simulink subsystem "Find_Target_Position_Velocity_Heading"  (R2023b)
settings: Solver=VariableStepAuto  StartTime=0.0  StopTime=10.0  RelTol=1e-3
undefined symbols (not defined in the file): Spline_Last_Pose_Distance_to_Velocity_Gain, Spline_Max_Centripital_Acceleration, Spline_Max_Num_RefPoses, Spline_Num_Samples, Spline_Pose_Num_Before_End_Reduce_Speed, Spline_Velocity_Multiplier_TEST
libraries: simulink x3
settings Model: Creator=ander  LastModifiedBy=ander

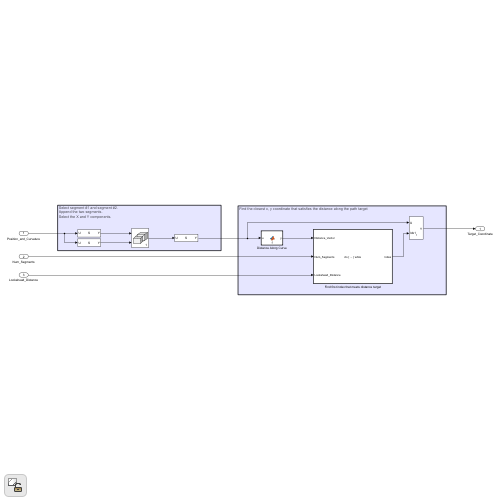
[thumbnail: Simulink's stored preview of the top-level diagram]
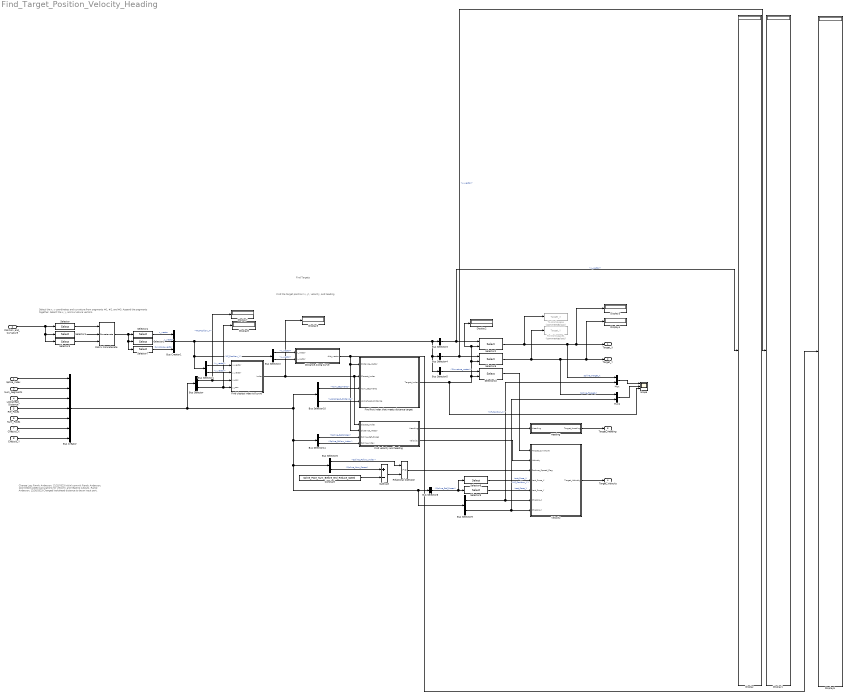
== system Find_Target_Position_Velocity_Heading ==
  note: Find the target position (x, y), velocity, and heading
  note: Select the x, y coordinates and curvature from segments #1, #2, and #3.
      | Append the segments together.
      | Select the x, y, and curvature vectors.
  note: Find Targets
  note: Change Log:
      | Randy Anderson: 12/25/2023
      | Initial commit
      | Randy Anderson, 12/27/2023
      | Added calculations for velocity and heading outputs.
      | Randy Anderson, 12/30/2023
      | Changed lookahead distance to be an input port.
  Spline_Index : Inport
  Position_and_Curvature : Inport  Port=2
  Num_Segments : Inport  Port=3
  Lookahead_Distance : Inport  Port=4  OutDataTypeStr=double  PortDimensions=1
  Ref_Poses : Inport  Port=5  OutDataTypeStr=double
  Num_Poses : Inport  Port=6
  Chassis_X : Inport  Port=7  OutDataTypeStr=double  PortDimensions=1
  Chassis_Y : Inport  Port=8  OutDataTypeStr=double  PortDimensions=1
  Bus Creator : BusCreator  Inputs=7
  Bus Creator1 : BusCreator  Inputs=3
  Bus Selector : BusSelector  OutputSignals=KF_Position_X,KF_Position_Y
  Bus Selector1 : BusSelector  OutputSignals=x_vector,y_vector
  Bus Selector10 : BusSelector  OutputSignals=Num_Segments,Lookahead_Distance
  Bus Selector11 : BusSelector  OutputSignals=Spline_Ref_Poses,Spline_Follow_Index
  Bus Selector2 : BusSelector  OutputSignals=x_vector,y_vector
  Bus Selector3 : BusSelector  OutputSignals=x_vector
  Bus Selector4 : BusSelector  OutputSignals=y_vector
  Bus Selector5 : BusSelector  OutputSignals=Curvature_vector
  Bus Selector6 : BusSelector  OutputSignals=Spline_Follow_Index,Spline_Num_Poses
  Bus Selector8 : BusSelector  OutputSignals=Spline_Ref_Poses
  Bus Selector9 : BusSelector  OutputSignals=KF_Position_X,KF_Position_Y
  Constant : Constant  Value=Spline_Pose_Num_Before_End_Reduce_Speed
  Display{,1..8} (9 alike) : Display
  Distance Along Curve : MATLAB Function  TreatAsAtomicUnit=on
  Find closest index to curve : MATLAB Function  TreatAsAtomicUnit=on
  Find first index that meets distance target : Subsystem  TreatAsAtomicUnit=on
  Find velocity and heading : Subsystem
  Heading : Subsystem
  Matrix Concatenate : Concatenate  NumInputs=3  Mode=Multidimensional array
  Mux : Mux  Inputs=2
  Mux1 : Mux  Inputs=2
  Relational Operator : RelationalOperator  OutDataTypeStr=boolean  RndMeth=Simplest  InputSameDT=off
  Scope : Scope  NumInputPorts=3
  Selector : Selector  NumberOfDimensions=3  InputPortWidth=3  IndexOptions=Select all,Select all,Index vector (dialog)  Indices=[1 3],[1 2],1  OutputSizes=1,1,1
  Selector1 : Selector  NumberOfDimensions=3  InputPortWidth=3  IndexOptions=Select all,Select all,Index vector (dialog)  Indices=[1 3],[1 2],2  OutputSizes=1,1,1
  Selector10 : Selector  InputPortWidth=Spline_Num_Samples_3x  IndexOptions=Index vector (port)  Indices=[1 3]  OutputSizes=1
  Selector2 : Selector  InputPortWidth=Spline_Num_Samples_3x  IndexOptions=Index vector (port)  Indices=[1 3]  OutputSizes=1
  Selector3 : Selector  NumberOfDimensions=3  InputPortWidth=3  IndexOptions=Select all,Select all,Index vector (dialog)  Indices=[1 3],[1 2],3  OutputSizes=1,1,1
  Selector4 : Selector  NumberOfDimensions=2  InputPortWidth=3  IndexOptions=Select all,Index vector (dialog)  Indices=[1 3],1  OutputSizes=1,1
  Selector5 : Selector  NumberOfDimensions=2  InputPortWidth=3  IndexOptions=Select all,Index vector (dialog)  Indices=[1 3],2  OutputSizes=1,1
  Selector6 : Selector  InputPortWidth=Spline_Num_Samples_3x  IndexOptions=Index vector (port)  Indices=[1 3]  OutputSizes=1
  Selector7 : Selector  NumberOfDimensions=2  InputPortWidth=3  IndexOptions=Select all,Index vector (dialog)  Indices=[1 3],3  OutputSizes=1,1
  Selector8 : Selector  NumberOfDimensions=2  InputPortWidth=3  IndexOptions=Index vector (dialog),Index vector (dialog)  Indices=Spline_Max_Num_RefPoses,1  OutputSizes=1,1
  Selector9 : Selector  NumberOfDimensions=2  InputPortWidth=3  IndexOptions=Index vector (dialog),Index vector (dialog)  Indices=Spline_Max_Num_RefPoses,2  OutputSizes=1,1
  Subtract : Sum  Inputs=+-
  To Workspace : ToWorkspace  Commented=on  VariableName=Target_X  SampleTime=-1
  To Workspace1 : ToWorkspace  Commented=on  VariableName=Target_Y  SampleTime=-1
  Velocity : Subsystem
  Target_X : Outport
  Target_Y : Outport  Port=2
  Target_Heading : Outport  Port=3
  Target_Velocity : Outport  Port=4
  wires:
  Selector1/1 -> Matrix Concatenate/2
  Matrix Concatenate/1 -> Selector4/1, Selector5/1, Selector7/1
  Selector/1 -> Matrix Concatenate/1
  Distance Along Curve/1(dist_vector) -> Find first index that meets distance target/1(Distance_Vector), Find velocity and heading/2(Distance_Vector), Display6/1
  Selector3/1 -> Matrix Concatenate/3
  Bus Creator/1 -> Bus Selector11/1, Bus Selector9/1, Bus Selector8/1, Bus Selector6/1, Bus Selector10/1, Bus Selector/1
  Selector5/1 -> Bus Creator1/2  "y_vector"
  Selector4/1 -> Bus Creator1/1  "x_vector"
  Bus Creator1/1 -> Bus Selector3/1, Bus Selector4/1, Bus Selector5/1, Bus Selector2/1, Bus Selector1/1
  Bus Selector1/1 -> Find closest index to curve/1(x_vector)  "<x_vector>"
  Bus Selector1/2 -> Find closest index to curve/2(y_vector)  "<y_vector>"
  Bus Selector/2 -> Find closest index to curve/4(y_pos), Display8/1  "<KF_Position_Y>"
  Bus Selector/1 -> Find closest index to curve/3(x_pos), Display7/1  "<KF_Position_X>"
  Bus Selector2/2 -> Distance Along Curve/2(y_vector)  "<y_vector>"
  Bus Selector2/1 -> Distance Along Curve/1(x_vector)  "<x_vector>"
  Bus Selector3/1 -> Selector2/1, Display/1  "<x_vector>"
  Bus Selector4/1 -> Selector6/1, Display1/1  "<y_vector>"
  Selector2/1 -> To Workspace/1, Target_X/1, Display3/1, Mux/1  "Spline_Target_X"
  Selector6/1 -> To Workspace1/1, Target_Y/1, Display4/1, Mux1/1  "Spline_Target_Y"
  Bus Selector10/2 -> Find first index that meets distance target/4(Lookahead_Distance)  "<Lookahead_Distance>"
  Position_and_Curvature/1 -> Selector/1, Selector1/1, Selector3/1
  Selector10/1 -> Velocity/1(Target_Curvature)
  Bus Selector5/1 -> Selector10/1  "<Curvature_vector>"
  Find first index that meets distance target/1(Target_Index) -> Display2/1, Selector2/2, Selector6/2, Selector10/2, Scope/3
  Selector7/1 -> Bus Creator1/3  "Curvature_vector"
  Constant/1 -> Subtract/2
  Subtract/1 -> Relational Operator/2
  Selector8/1 -> Velocity/4(Last_Pose_X)  "Last_Pose_X"
  Selector9/1 -> Velocity/5(Last_Pose_Y)  "Last_Pose_Y"
  Relational Operator/1 -> Velocity/3(Reduce_Speed_Flag)
  Velocity/1(Target_Velocity) -> Target_Velocity/1
  Bus Selector6/1 -> Relational Operator/1  "<Spline_Follow_Index>"
  Bus Selector8/1 -> Selector9/1, Selector8/1  "<Spline_Ref_Poses>"
  Bus Selector9/1 -> Velocity/6(Chassis_X), Mux/2  "<KF_Position_X>"
  Bus Selector9/2 -> Velocity/7(Chassis_Y), Mux1/2  "<KF_Position_Y>"
  Bus Selector10/1 -> Find first index that meets distance target/3(Num_Segments)  "<Num_Segments>"
  Spline_Index/1 -> Bus Creator/1
  Num_Segments/1 -> Bus Creator/2
  Ref_Poses/1 -> Bus Creator/4
  Num_Poses/1 -> Bus Creator/5
  Chassis_X/1 -> Bus Creator/6
  Chassis_Y/1 -> Bus Creator/7
  Heading/1(Target_Heading) -> Target_Heading/1
  Bus Selector6/2 -> Subtract/1  "<Spline_Num_Poses>"
  Find closest index to curve/1(index) -> Find first index that meets distance target/2(Closest_Index), Find velocity and heading/1(Closest_Index), Display5/1
  Bus Selector11/1 -> Find velocity and heading/3(Spline_Ref_Poses)  "<Spline_Ref_Poses>"
  Bus Selector11/2 -> Find velocity and heading/4(Spline_Index)  "<Spline_Follow_Index>"
  Find velocity and heading/2(Velocity) -> Velocity/2(Velocity)
  Find velocity and heading/1(Heading) -> Heading/1(Heading)
  Lookahead_Distance/1 -> Bus Creator/3
  Mux/1 -> Scope/1
  Mux1/1 -> Scope/2

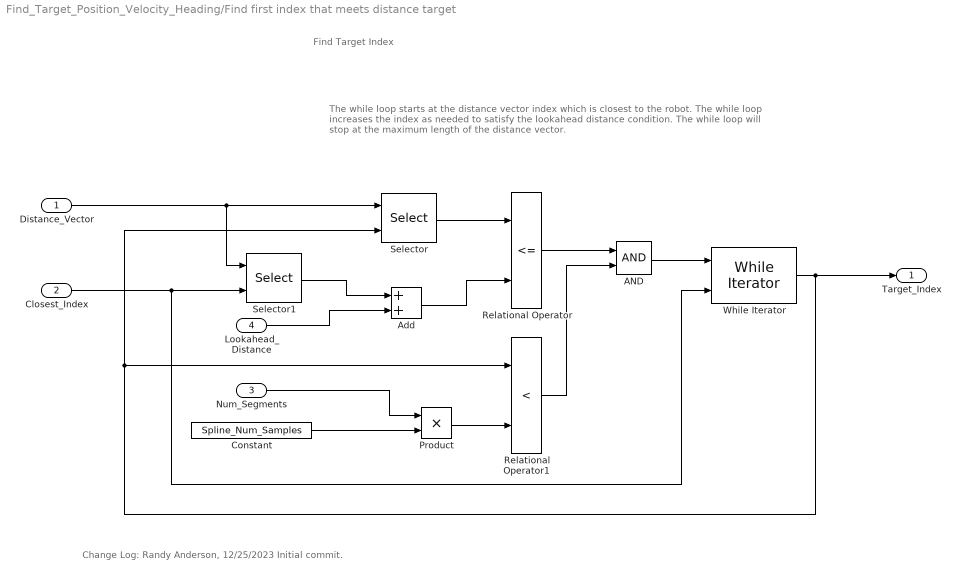
== system Find_Target_Position_Velocity_Heading/Find first index that meets distance target ==
  note: Change Log:
      | Randy Anderson, 12/25/2023
      | Initial commit.
  note: The while loop starts at the distance vector index which is closest to the robot.
      | The while loop increases the index as needed to satisfy the lookahead distance condition.
      | The while loop will stop at the maximum length of the distance vector.
  note: Find Target Index
  Distance_Vector : Inport
  Closest_Index : Inport  Port=2
  Num_Segments : Inport  Port=3
  Lookahead_Distance : Inport  Port=4
  AND : Logic  AllPortsSameDT=off  OutDataTypeStr=boolean
  Add : Sum
  Constant : Constant  Value=Spline_Num_Samples
  Product : Product
  Relational Operator : RelationalOperator  Operator=<=  OutDataTypeStr=boolean  RndMeth=Simplest  InputSameDT=off
  Relational Operator1 : RelationalOperator  Operator=<  OutDataTypeStr=boolean  RndMeth=Simplest  InputSameDT=off
  Selector : Selector  InputPortWidth=Spline_Num_Samples_3x  IndexOptions=Index vector (port)  Indices=[1 3]  OutputSizes=1
  Selector1 : Selector  InputPortWidth=Spline_Num_Samples_3x  IndexOptions=Index vector (port)  Indices=[1 3]  OutputSizes=1
  While Iterator : WhileIterator  MaxIters=Spline_Num_Samples_3x  ShowIterationPort=on  OutputDataType=uint16
  Target_Index : Outport
  wires:
  Selector1/1 -> Add/1
  Lookahead_Distance/1 -> Add/2
  Add/1 -> Relational Operator/2
  Closest_Index/1 -> Selector1/2, While Iterator/2
  AND/1 -> While Iterator/1
  Relational Operator/1 -> AND/1
  Relational Operator1/1 -> AND/2
  Constant/1 -> Product/2
  Num_Segments/1 -> Product/1
  Product/1 -> Relational Operator1/2
  While Iterator/1 -> Selector/2, Relational Operator1/1, Target_Index/1
  Selector/1 -> Relational Operator/1
  Distance_Vector/1 -> Selector/1, Selector1/1

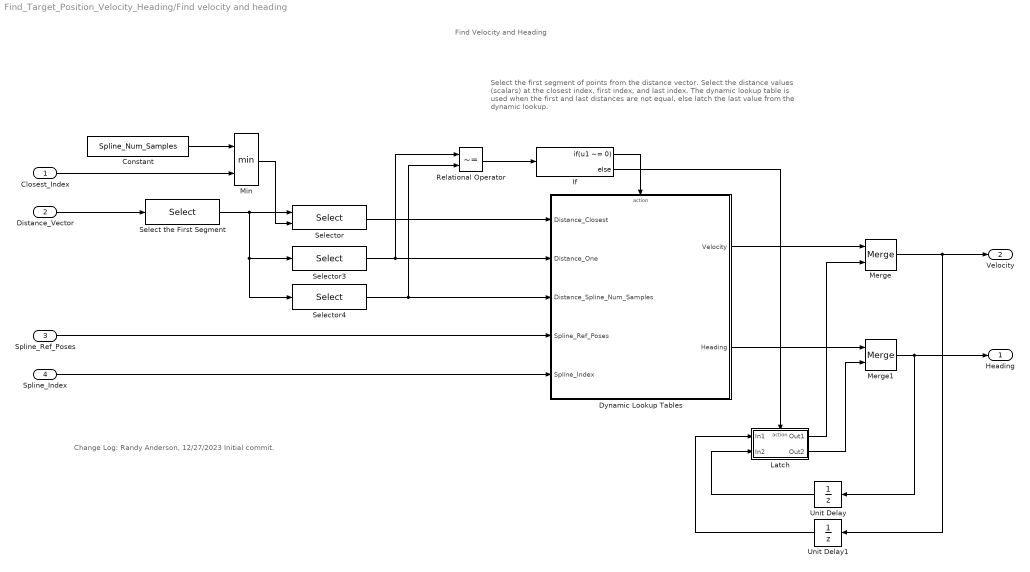
== system Find_Target_Position_Velocity_Heading/Find velocity and heading ==
  note: Change Log:
      | Randy Anderson, 12/27/2023
      | Initial commit.
  note: Find Velocity and Heading
  note: Select the first segment of points from the distance vector.
      | Select the distance values (scalars) at the closest index, first index, and last index.
      | The dynamic lookup table is used when the first and last distances are not equal,
      |    else latch the last value from the dynamic lookup.
  Closest_Index : Inport
  Distance_Vector : Inport  Port=2
  Spline_Ref_Poses : Inport  Port=3
  Spline_Index : Inport  Port=4
  Constant : Constant  Value=Spline_Num_Samples
  Dynamic Lookup Tables : Subsystem
  If : If  IfExpression=u1 ~= 0
  Latch : Subsystem  TreatAsAtomicUnit=on
  Merge : Merge
  Merge1 : Merge
  Min : MinMax  Inputs=2
  Relational Operator : RelationalOperator  Operator=~=  OutDataTypeStr=boolean  RndMeth=Simplest  InputSameDT=off
  Select the First Segment : Selector  InputPortWidth=Spline_Num_Samples_3x  IndexOptions=Index vector (dialog)  Indices=[1:Spline_Num_Samples]  OutputSizes=1
  Selector : Selector  InputPortWidth=Spline_Num_Samples  IndexOptions=Index vector (port)  Indices=[1:Spline_Num_Samples]  OutputSizes=1
  Selector3 : Selector  InputPortWidth=Spline_Num_Samples  IndexOptions=Index vector (dialog)  Indices=1  OutputSizes=1
  Selector4 : Selector  InputPortWidth=Spline_Num_Samples  IndexOptions=Index vector (dialog)  Indices=Spline_Num_Samples  OutputSizes=1
  Unit Delay : UnitDelay  SampleTime=-1  HasFrameUpgradeWarning=on
  Unit Delay1 : UnitDelay  SampleTime=-1  HasFrameUpgradeWarning=on
  Heading : Outport
  Velocity : Outport  Port=2
  wires:
  Constant/1 -> Min/1
  Min/1 -> Selector/2
  Unit Delay1/1 -> Latch/1(In1)
  Unit Delay/1 -> Latch/2(In2)
  Merge/1 -> Velocity/1, Unit Delay1/1
  Merge1/1 -> Unit Delay/1, Heading/1
  Latch/2(Out2) -> Merge1/2
  Dynamic Lookup Tables/2(Heading) -> Merge1/1
  Latch/1(Out1) -> Merge/2
  Dynamic Lookup Tables/1(Velocity) -> Merge/1
  If/2 -> Latch/Action
  If/1 -> Dynamic Lookup Tables/Action
  Spline_Index/1 -> Dynamic Lookup Tables/5(Spline_Index)
  Spline_Ref_Poses/1 -> Dynamic Lookup Tables/4(Spline_Ref_Poses)
  Selector/1 -> Dynamic Lookup Tables/1(Distance_Closest)
  Relational Operator/1 -> If/1
  Selector4/1 -> Dynamic Lookup Tables/3(Distance_Spline_Num_Samples), Relational Operator/2
  Select the First Segment/1 -> Selector/1, Selector3/1, Selector4/1
  Selector3/1 -> Dynamic Lookup Tables/2(Distance_One), Relational Operator/1
  Closest_Index/1 -> Min/2
  Distance_Vector/1 -> Select the First Segment/1

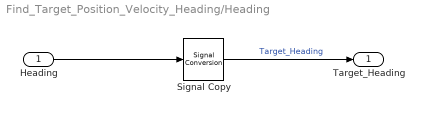
== system Find_Target_Position_Velocity_Heading/Heading ==
  Heading : Inport
  Signal Copy : SignalConversion  OverrideOpt=off
  Target_Heading : Outport
  wires:
  Heading/1 -> Signal Copy/1
  Signal Copy/1 -> Target_Heading/1  "Target_Heading"

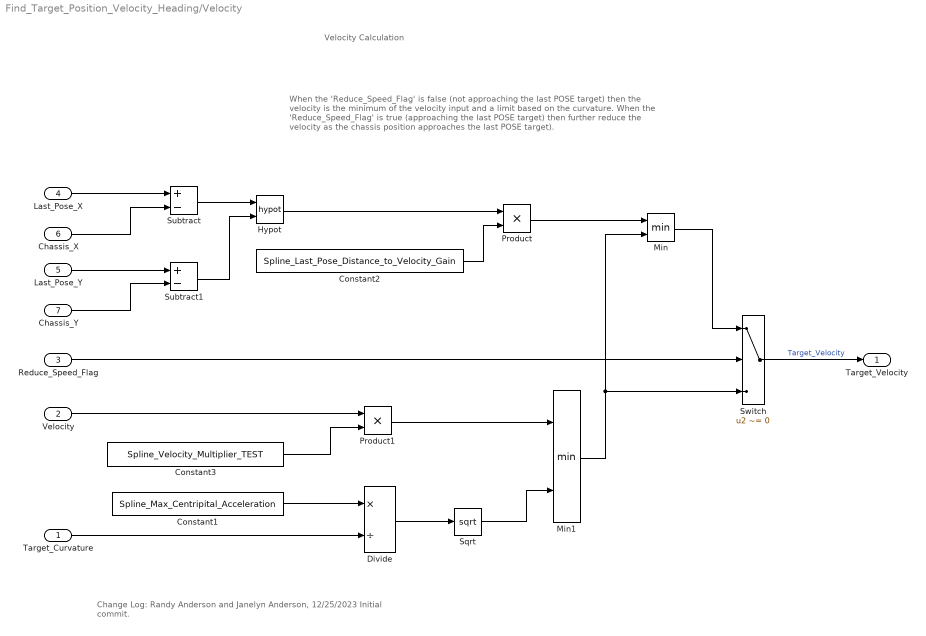
== system Find_Target_Position_Velocity_Heading/Velocity ==
  note: When the 'Reduce_Speed_Flag' is false (not approaching the last POSE target) then
      | the velocity is the minimum of the velocity input and a limit based on the curvature.
      |
      | When the 'Reduce_Speed_Flag' is true (approaching the last POSE target) then further
      | reduce the velocity as the chassis position approaches the last POSE target).
  note: Velocity Calculation
  note: Change Log:
      | Randy Anderson and Janelyn Anderson, 12/25/2023
      | Initial commit.
  Target_Curvature : Inport
  Velocity : Inport  Port=2
  Reduce_Speed_Flag : Inport  Port=3
  Last_Pose_X : Inport  Port=4
  Last_Pose_Y : Inport  Port=5
  Chassis_X : Inport  Port=6  OutDataTypeStr=double  PortDimensions=1
  Chassis_Y : Inport  Port=7  OutDataTypeStr=double  PortDimensions=1
  Constant1 : Constant  Value=Spline_Max_Centripital_Acceleration
  Constant2 : Constant  Value=Spline_Last_Pose_Distance_to_Velocity_Gain
  Constant3 : Constant  Value=Spline_Velocity_Multiplier_TEST
  Divide : Product  Inputs=*/
  Hypot : Math  Operator=hypot
  Min : MinMax  Inputs=2
  Min1 : MinMax  Inputs=2
  Product : Product
  Product1 : Product
  Sqrt : Sqrt
  Subtract : Sum  Inputs=+-
  Subtract1 : Sum  Inputs=+-
  Switch : Switch  Criteria=u2 ~= 0  SaturateOnIntegerOverflow=off  InputSameDT=off
  Target_Velocity : Outport
  wires:
  Constant3/1 -> Product1/2
  Velocity/1 -> Product1/1
  Product1/1 -> Min1/1
  Switch/1 -> Target_Velocity/1  "Target_Velocity"
  Constant2/1 -> Product/2
  Product/1 -> Min/1
  Hypot/1 -> Product/1
  Sqrt/1 -> Min1/2
  Divide/1 -> Sqrt/1
  Constant1/1 -> Divide/1
  Target_Curvature/1 -> Divide/2
  Min/1 -> Switch/1
  Reduce_Speed_Flag/1 -> Switch/2
  Min1/1 -> Switch/3, Min/2
  Subtract1/1 -> Hypot/2
  Subtract/1 -> Hypot/1
  Chassis_Y/1 -> Subtract1/2
  Last_Pose_Y/1 -> Subtract1/1
  Chassis_X/1 -> Subtract/2
  Last_Pose_X/1 -> Subtract/1

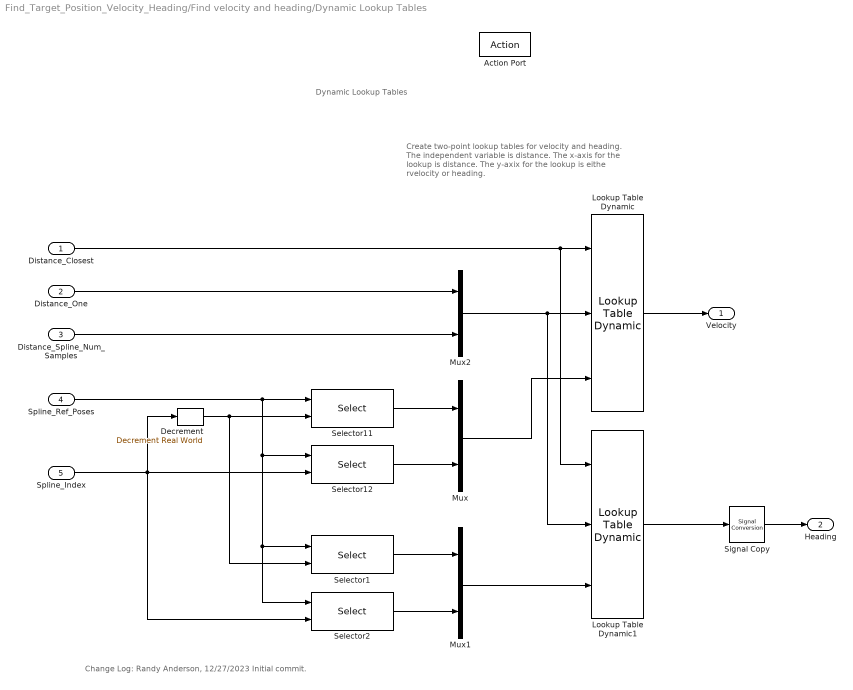
== system Find_Target_Position_Velocity_Heading/Find velocity and heading/Dynamic Lookup Tables ==
  note: Change Log:
      | Randy Anderson, 12/27/2023
      | Initial commit.
  note: Dynamic Lookup Tables
  note: Create two-point lookup tables for velocity and heading.
      | The independent variable is distance.
      | The x-axis for the lookup is distance.
      | The y-axix for the lookup is eithe rvelocity or heading.
  Distance_Closest : Inport
  Distance_One : Inport  Port=2
  Distance_Spline_Num_Samples : Inport  Port=3
  Spline_Ref_Poses : Inport  Port=4
  Spline_Index : Inport  Port=5
  Action Port : ActionPort
  Decrement : simulink/Additional Math & Discrete/Additional Math: Increment - Decrement/Decrement Real World
  Lookup Table Dynamic : simulink/Lookup Tables/Lookup Table Dynamic  LookUpMeth=Interpolation-Use End Values  OutDataType=fixdt('double')  OutScaling=[]  OutputDataTypeScalingMode=Specify via dialog  OutDataTypeStr=double  DoSatur=off
  Lookup Table Dynamic1 : simulink/Lookup Tables/Lookup Table Dynamic  LookUpMeth=Interpolation-Use End Values  OutDataType=fixdt('double')  OutScaling=[]  OutputDataTypeScalingMode=Specify via dialog  OutDataTypeStr=double  DoSatur=off
  Mux : Mux  Inputs=2
  Mux1 : Mux  Inputs=2
  Mux2 : Mux  Inputs=2
  Selector1 : Selector  NumberOfDimensions=2  InputPortWidth=Spline_Num_Samples_x3  IndexOptions=Index vector (port),Index vector (dialog)  Indices=[1 3],4  OutputSizes=1,1
  Selector11 : Selector  NumberOfDimensions=2  InputPortWidth=Spline_Num_Samples_x3  IndexOptions=Index vector (port),Index vector (dialog)  Indices=[1 3],3  OutputSizes=1,1
  Selector12 : Selector  NumberOfDimensions=2  InputPortWidth=Spline_Num_Samples_x3  IndexOptions=Index vector (port),Index vector (dialog)  Indices=[1 3],3  OutputSizes=1,1
  Selector2 : Selector  NumberOfDimensions=2  InputPortWidth=Spline_Num_Samples_x3  IndexOptions=Index vector (port),Index vector (dialog)  Indices=[1 3],4  OutputSizes=1,1
  Signal Copy : SignalConversion  OverrideOpt=off
  Velocity : Outport
  Heading : Outport  Port=2
  wires:
  Signal Copy/1 -> Heading/1
  Mux/1 -> Lookup Table Dynamic/3
  Distance_One/1 -> Mux2/1
  Lookup Table Dynamic/1 -> Velocity/1
  Selector1/1 -> Mux1/1
  Selector11/1 -> Mux/1
  Distance_Spline_Num_Samples/1 -> Mux2/2
  Decrement/1 -> Selector1/2, Selector11/2
  Mux1/1 -> Lookup Table Dynamic1/3
  Selector2/1 -> Mux1/2
  Mux2/1 -> Lookup Table Dynamic/2, Lookup Table Dynamic1/2
  Spline_Index/1 -> Selector12/2, Selector2/2, Decrement/1
  Lookup Table Dynamic1/1 -> Signal Copy/1
  Spline_Ref_Poses/1 -> Selector12/1, Selector1/1, Selector2/1, Selector11/1
  Selector12/1 -> Mux/2
  Distance_Closest/1 -> Lookup Table Dynamic/1, Lookup Table Dynamic1/1

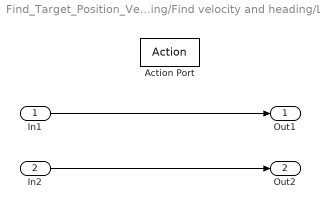
== system Find_Target_Position_Velocity_Heading/Find velocity and heading/Latch ==
  In1 : Inport
  In2 : Inport  Port=2
  Action Port : ActionPort
  Out1 : Outport
  Out2 : Outport  Port=2
  wires:
  In2/1 -> Out2/1
  In1/1 -> Out1/1

== matlab function Find_Target_Position_Velocity_Heading/Distance Along Curve ==
  data: x_vector input; dist_vector output; y_vector input
function dist_vector = distance(x_vector,y_vector)
% Calculate the distance vector along the curve x, y coordinate pair
% from the first index to the last index.
%
% Randy Anderson
% 2023-12-21

len = length(x_vector);
dist_vector = zeros(len,1);
for k = 2:len
    x_delta = x_vector(k)-x_vector(k-1);
    y_delta = y_vector(k)-y_vector(k-1);
    distance = hypot(x_delta,y_delta);
    dist_vector(k) = dist_vector(k-1) + distance;
end

== matlab function Find_Target_Position_Velocity_Heading/Find closest index to curve ==
  data: x_vector input; index output; y_vector input; x_pos input; y_pos input
function index = find_index(x_vector,y_vector,x_pos,y_pos)
% Finds the index corresponding to input x, y vectors that is the closest
% coordinate pair along the curve to the robot x, y position.
%
% Randy Anderson
% 2023-12-23

len = length(x_vector);
distance_from_robot = zeros(len,1);
for k = 1:len
    x_delta = x_vector(k)-x_pos;
    y_delta = y_vector(k)-y_pos;
    distance_from_robot(k) = hypot(x_delta,y_delta);
end

min_distance = min(distance_from_robot);

for k = 1:len
    if distance_from_robot(k) == min_distance
        break
    end
end

index = k;
